simulink model "Zeitdiskrete_PT1_Glied_simu"  (Simulink 7.3)
settings: Solver=ode45  StartTime=0.0  StopTime=2  RelTol=1e-3
values from neighbouring files (symbols this model uses):
  T = 0.1    [Zeitdiskrete_PT1_Glied.m]
  Ta = 0.01*tend    (= 0.05)    [Zeitdiskrete_PT1_Glied.m]
libraries: simulink x1
settings Model: Creator=Juan Duran  LastModifiedBy=Juan Duran

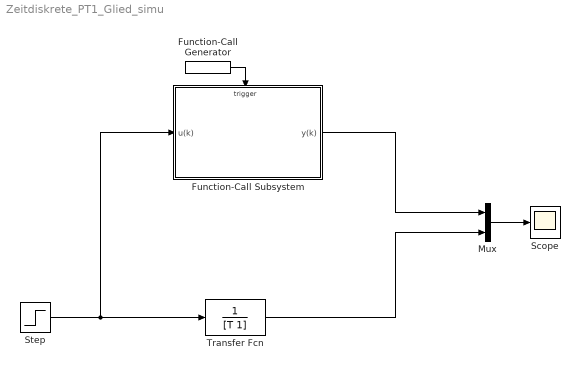
== system Zeitdiskrete_PT1_Glied_simu ==
  Function-Call Generator : simulink/Ports & Subsystems/Function-Call Generator  sample_time=Ta  numberOfIterations=1
  Function-Call Subsystem : Subsystem  TreatAsAtomicUnit=on
  Mux : Mux  Inputs=2
  Scope : Scope
  Step : Step  SampleTime=0
  Transfer Fcn : TransferFcn  Denominator=[T 1]
  wires:
  Step/1 -> Transfer Fcn/1, Function-Call Subsystem/1(u(k))
  Function-Call Generator/1 -> Function-Call Subsystem/Trigger
  Function-Call Subsystem/1(y(k)) -> Mux/1
  Transfer Fcn/1 -> Mux/2
  Mux/1 -> Scope/1

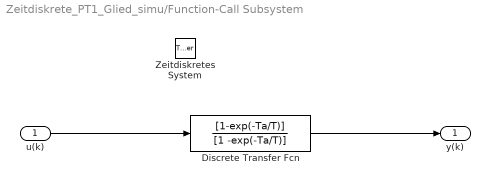
== system Zeitdiskrete_PT1_Glied_simu/Function-Call Subsystem ==
  u(k) : Inport  OutDataType=fixdt(1, 16)  OutScaling=2^0
  Zeitdiskretes System : TriggerPort  TriggerType=function-call
  Discrete Transfer Fcn : DiscreteTransferFcn  Numerator=[1-exp(-Ta/T)]  Denominator=[1 -exp(-Ta/T)]  SampleTime=-1
  y(k) : Outport  OutDataType=fixdt(1, 16)  OutScaling=2^0
  wires:
  u(k)/1 -> Discrete Transfer Fcn/1
  Discrete Transfer Fcn/1 -> y(k)/1
